simulink model "experiment2"  (R2020a)
settings: Solver=ode4  StartTime=0.0  StopTime=5  FixedStep=0.0001  RelTol=1e-3
values from neighbouring files (symbols this model uses):
  A = lstm1_getContinuousA(I_zz,c_alpha_fl,c_alpha_fr,c_alpha_rl,c_alpha_rr,l_f,l_r,m,v)    [run_experiment.m]
  Ad = sysd.a    [run_experiment.m]
  B = lstm1_getContinuousB(I_zz,c_alpha_fl,c_alpha_fr,c_alpha_rl,c_alpha_rr,l_f,l_r,m,v)    [run_experiment.m]
  Bd = sysd.b(:,1:3)    [run_experiment.m]
  C = [C_psi_dot;C_ay]    [run_experiment.m]
  Cd = sysd.c    [run_experiment.m]
  D = [D_psi_dot;D_ay]    [run_experiment.m]
  Dd = sysd.d(:,1:3)    [run_experiment.m]
  G = eye(noise_process_cnt)    [run_experiment.m]
  Gd = sysd.b(:,4:3+noise_process_cnt)    [run_experiment.m]
  Q_chol = chol(Q_real)    [run_experiment.m]
  R_chol = chol(R_real)    [run_experiment.m]
  td = 0.001    [run_experiment.m]
  x0 = lstm1_buildX(psi_dot,beta)    [run_experiment.m]
settings Model: Creator=danie  LastModifiedBy=danie

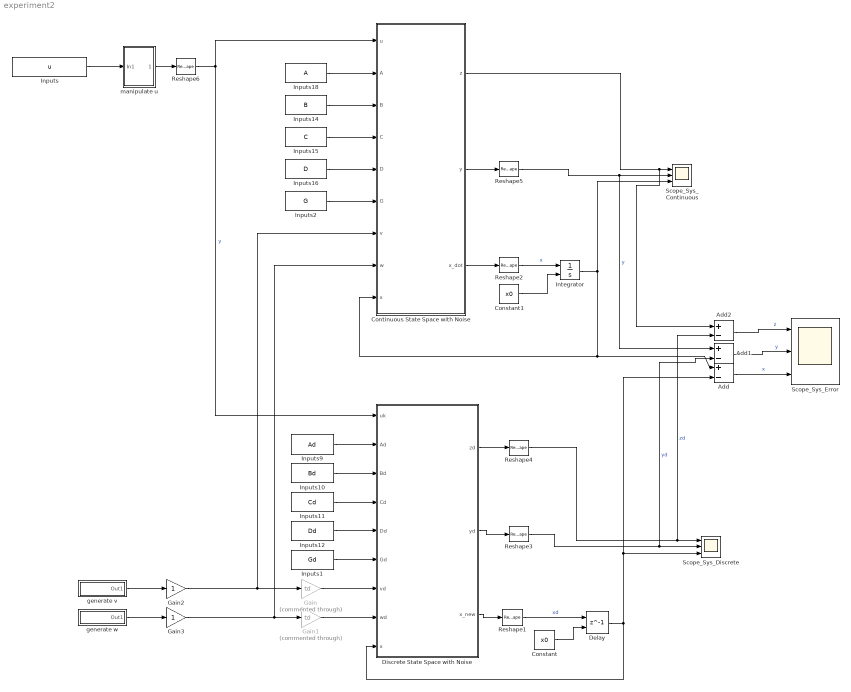
== system experiment2 ==
  Add : Sum  Inputs=+-
  Add1 : Sum  Inputs=+-
  Add2 : Sum  Inputs=+-
  Constant : Constant  Value=x0  VectorParams1D=off
  Constant1 : Constant  Value=x0  VectorParams1D=off
  Continuous State Space with Noise : MATLAB Function  TreatAsAtomicUnit=on
  Delay : Delay  DelayLength=1  InitialConditionSource=Input port  SampleTime=td
      settings: InputPortMap=u0,p4
  Discrete State Space with Noise : MATLAB Function  TreatAsAtomicUnit=on  SystemSampleTime=td
  Gain : Gain  Commented=through  Gain=td
  Gain1 : Gain  Commented=through  Gain=td
  Gain2 : Gain
  Gain3 : Gain
  Inputs : Constant  Value=u  VectorParams1D=off  SampleTime=td*2
  Inputs1 : Constant  Value=Gd  SampleTime=td
  Inputs10 : Constant  Value=Bd  SampleTime=td
  Inputs11 : Constant  Value=Cd  SampleTime=td
  Inputs12 : Constant  Value=Dd  SampleTime=td
  Inputs14 : Constant  Value=B  SampleTime=td
  Inputs15 : Constant  Value=C  SampleTime=td
  Inputs16 : Constant  Value=D  SampleTime=td
  Inputs18 : Constant  Value=A  SampleTime=td
  Inputs2 : Constant  Value=G  SampleTime=td
  Inputs9 : Constant  Value=Ad  SampleTime=td
  Integrator : Integrator  InitialConditionSource=external
  Reshape{1..6} (6 alike) : Reshape  OutputDimensionality=Column vector (2-D)
  Scope_Sys_Continuous : Scope  NumInputPorts=3
  Scope_Sys_Discrete : Scope  NumInputPorts=3
  Scope_Sys_Error : Scope  NumInputPorts=3
  generate v : Subsystem
  generate w : Subsystem
  manipulate u : Subsystem
  wires:
  Inputs12/1 -> Discrete State Space with Noise/5(Dd)
  Inputs11/1 -> Discrete State Space with Noise/4(Cd)
  Inputs10/1 -> Discrete State Space with Noise/3(Bd)
  Inputs9/1 -> Discrete State Space with Noise/2(Ad)
  Discrete State Space with Noise/1(zd) -> Reshape4/1
  Discrete State Space with Noise/2(yd) -> Reshape3/1
  Discrete State Space with Noise/3(x_new) -> Reshape1/1
  Reshape1/1 -> Delay/1  "xd"
  Constant/1 -> Delay/2
  Delay/1 -> Discrete State Space with Noise/9(x), Add/2, Scope_Sys_Discrete/3
  Reshape3/1 -> Add1/2, Scope_Sys_Discrete/2  "yd"
  Reshape4/1 -> Add2/2, Scope_Sys_Discrete/1  "zd"
  Inputs/1 -> manipulate u/1(In1)
  manipulate u/1(Out1) -> Reshape6/1
  Inputs1/1 -> Discrete State Space with Noise/6(Gd)
  Reshape6/1 -> Discrete State Space with Noise/1(uk), Continuous State Space with Noise/1(u)  "y"
  generate w/1(Out1) -> Gain3/1
  Inputs18/1 -> Continuous State Space with Noise/2(A)
  Inputs14/1 -> Continuous State Space with Noise/3(B)
  Inputs15/1 -> Continuous State Space with Noise/4(C)
  Inputs16/1 -> Continuous State Space with Noise/5(D)
  Inputs2/1 -> Continuous State Space with Noise/6(G)
  Constant1/1 -> Integrator/2
  Integrator/1 -> Add/1, Continuous State Space with Noise/9(x), Scope_Sys_Continuous/3
  Continuous State Space with Noise/3(x_dot) -> Reshape2/1
  Reshape2/1 -> Integrator/1  "x"
  generate v/1(Out1) -> Gain2/1
  Continuous State Space with Noise/2(y) -> Reshape5/1
  Continuous State Space with Noise/1(z) -> Add2/1, Scope_Sys_Continuous/1
  Reshape5/1 -> Add1/1, Scope_Sys_Continuous/2  "y"
  Gain2/1 -> Gain/1, Continuous State Space with Noise/7(v)
  Gain3/1 -> Gain1/1, Continuous State Space with Noise/8(w)
  Add/1 -> Scope_Sys_Error/3  "x"
  Add1/1 -> Scope_Sys_Error/2  "y"
  Add2/1 -> Scope_Sys_Error/1  "z"
  Gain/1 -> Discrete State Space with Noise/7(vd)
  Gain1/1 -> Discrete State Space with Noise/8(wd)

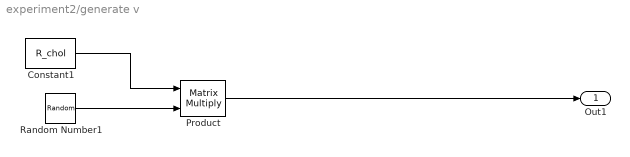
== system experiment2/generate v ==
  Constant1 : Constant  Value=R_chol  VectorParams1D=off
  Product : Product  Multiplication=Matrix(*)
  Random Number1 : RandomNumber  Mean=[0;0]  Variance=[1;1]  Seed=[0;1]  VectorParams1D=off
  Out1 : Outport
  wires:
  Random Number1/1 -> Product/2
  Constant1/1 -> Product/1
  Product/1 -> Out1/1

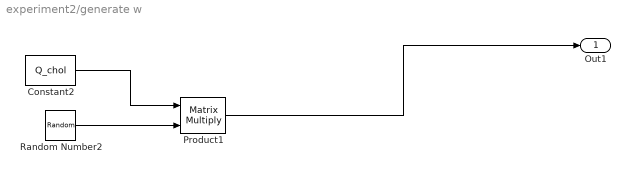
== system experiment2/generate w ==
  Constant2 : Constant  Value=Q_chol  VectorParams1D=off
  Product1 : Product  Multiplication=Matrix(*)
  Random Number2 : RandomNumber  Mean=[0;0]  Variance=[1;1]  Seed=[0;1]  VectorParams1D=off
  Out1 : Outport
  wires:
  Random Number2/1 -> Product1/2
  Product1/1 -> Out1/1
  Constant2/1 -> Product1/1

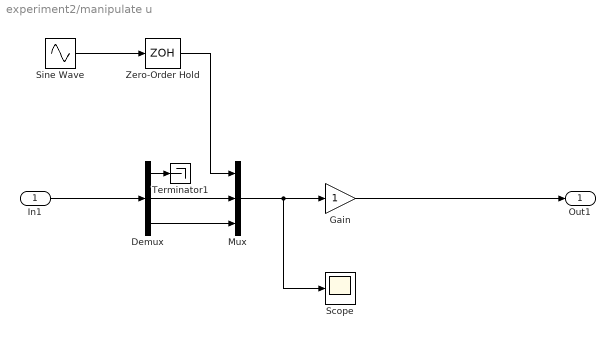
== system experiment2/manipulate u ==
  In1 : Inport
  Demux : Demux  Outputs=3
  Gain : Gain
  Mux : Mux  Inputs=3
  Scope : Scope
  Sine Wave : Sin  Amplitude=deg2rad(5)  SampleTime=0
  Terminator1 : Terminator
  Zero-Order Hold : ZeroOrderHold  SampleTime=0.1
  Out1 : Outport
  wires:
  In1/1 -> Demux/1
  Mux/1 -> Gain/1, Scope/1
  Sine Wave/1 -> Zero-Order Hold/1
  Gain/1 -> Out1/1
  Demux/2 -> Mux/2
  Demux/1 -> Terminator1/1
  Demux/3 -> Mux/3
  Zero-Order Hold/1 -> Mux/1

== matlab function experiment2/Discrete State Space with Noise ==
  data: zd output; yd output; x_new output; uk input; Ad input; Bd input; Cd input; Dd input; Gd input; vd input; wd input; x input
function [zd,yd,x_new]  = fcn(uk,Ad,Bd,Cd,Dd,Gd,vd,wd,x)
%%%%%%%%%%%%%%%%%%%%%%%%%%%%%%%%%%%%%%%%%%%%%%%%%%%%%%%%%%%%%%%%%%%%%%%%%%
% Author:       Daniel Ossig
% Date:         26.07.2018
%
% Description:
%
% MATLAB Vers.: 2017a
%
%%%%%%%%%%%%%%%%%%%%%%%%%%%%%%%%%%%%%%%%%%%%%%%%%%%%%%%%%%%%%%%%%%%%%%%%%%
%#codegen


x_new = Ad*x+Bd*uk+Gd*wd;
yd     = Cd*x+Dd*uk;
zd     = yd+vd;

== matlab function experiment2/Continuous State Space with Noise ==
  data: z output; y output; u input; A input; B input; C input; D input; G input; v input; w input; x input; x_dot output
function [z,y,x_dot]  = fcn(u,A,B,C,D,G,v,w,x)
%%%%%%%%%%%%%%%%%%%%%%%%%%%%%%%%%%%%%%%%%%%%%%%%%%%%%%%%%%%%%%%%%%%%%%%%%%
% Author:       Daniel Ossig
% Date:         26.07.2018
%
% Description:
%
% MATLAB Vers.: 2017a
%
%%%%%%%%%%%%%%%%%%%%%%%%%%%%%%%%%%%%%%%%%%%%%%%%%%%%%%%%%%%%%%%%%%%%%%%%%%
%#codegen


x_dot = A*x+B*u+G*w;
y     = C*x+D*u;
z     = y+v;
